simulink model "P0706"  (Simulink 10.2)
settings: Solver=VariableStepDiscrete  StartTime=0.0  StopTime=1  MaxStep=1  RelTol=1e-3
settings Model: Creator=Ranci  LastModifiedBy=Ranci
settings DataIOCC: SaveFormat=Dataset  SignalLoggingSaveFormat=Dataset  ReturnWorkspaceOutputs=on
settings OptimizationCC: LifeSpan=auto
settings DebuggingCC: UnderspecifiedInitializationDetection=Simplified  MergeDetectMultiDrivingBlocksExec=error  FcnCallInpInsideContextMsg=error  SFUnexpectedBacktrackingDiag=error  SFNoUnconditionalDefaultTransitionDiag=error  SFExecutionAtInitializationDiag=warning  ArithmeticOperatorsInVariantConditions=error
settings HardwareCC: ProdBitPerPointer=64  ProdBitPerSizeT=64  ProdBitPerPtrDiffT=64  ProdLargestAtomicFloat=Float  ProdIntDivRoundTo=Zero  ProdEndianess=LittleEndian  ProdWordSize=64  ProdHWDeviceType=Intel->x86-64 (Windows64)
settings ModelReferenceCC: PropagateSignalLabelsOutOfModel=on
settings SFSimCC: SimUseLocalCustomCode=on  CustomCodeUndefinedFunction=FilterOut
settings RTWCC: RTWUseLocalCustomCode=on
settings CodeAppCC: StateflowObjectComments=off
settings GRTTargetCC: TargetLangStandard=C99 (ISO)  CombineOutputUpdateFcns=on  GRTInterface=off
settings ConfigComp: CovMetricSettings=dwe  CovSaveCumulativeToWorkspaceVar=off  CovSaveSingleToWorkspaceVar=off  CovExternalEMLEnable=on

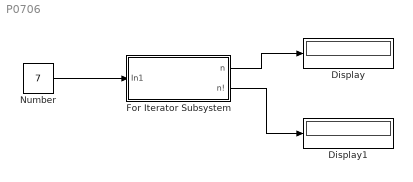
== system P0706 ==
  Display : Display
  Display1 : Display
  For Iterator Subsystem : Subsystem  TreatAsAtomicUnit=on
  Number : Constant  Value=7
  wires:
  Number/1 -> For Iterator Subsystem/1(In1)
  For Iterator Subsystem/1(n) -> Display/1
  For Iterator Subsystem/2(n!) -> Display1/1

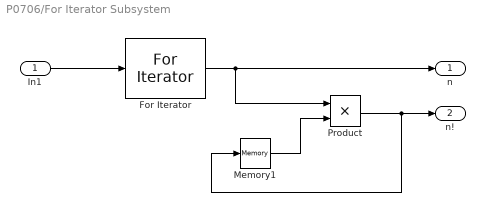
== system P0706/For Iterator Subsystem ==
  In1 : Inport
  For Iterator : ForIterator  ResetStates=reset  IterationSource=external
  Memory1 : Memory  InitialCondition=1  InheritSampleTime=on
  Product : Product  OutDataTypeStr=int64
  n : Outport
  n! : Outport  Port=2
  wires:
  In1/1 -> For Iterator/1
  For Iterator/1 -> Product/1, n/1
  Product/1 -> Memory1/1, n!/1
  Memory1/1 -> Product/2
